simulink model "Multibody_model_El_winch"  (R2023b)
settings: Solver=FixedStepAuto  StartTime=0.0  StopTime=25  FixedStep=0.001  RelTol=1e-3
model workspace (MATLAB code in the model file):
  | % Parameters
  | Q_max = 130; %L/min |  2 vales w max 65 L/min
  | 
  | %Load Parameters
  | m_pl = 1000;
  | r_d = 0.035;
  | ig = 5;
  | J_drum = 0.0006125; % 1/2MR^2
  | b_hat = 0.001;
  | 
  | % Motor Parameters
  | np=2;
  | P_N = 15000;
  | n_eff = 0.917;
  | n_rpm = 1469;
  | pf = 0.84;
  | I_N = 29;
  | Is_In = 8;
  | T_n = 97.5;
  | Ti_Tn = 3.1;
  | Tb_Tn = 3.6;
  | J_motor = 0.13;
  | 
  | % Inv-Gamma Circuit parameters
  | 
  | R_R_hat = 0.2052;
  | X_M_opt = 15.1061;
  | X_sig_opt = 0.3774;
  | omega_rN = 307.6666;
  | omega_N = 314.1593;
  | omega1 = omega_rN;
  | L_M_hat = X_M_opt/omega1;
  | L_sig_hat = X_sig_opt/omega1;
  | R_s = 0.619;
  | 
  | 
  | psi_ref = 20*P_N/(sqrt(2)*pi*np*I_N*n_rpm);
  | 
  | % Others
  | V_base = 400*sqrt(2)/sqrt(3);
  | I_max = I_N*3;
  | 
  | % Speed Controller
  | t_r = 1e-3;
  | w_BW = log(9)/t_r;
  | w_BWs = 0.1*w_BW;
  | J_hat = m_pl*((r_d/(ig))^2) + J_drum*((1/ig)^2) + J_motor;
  | kps = 2*J_hat*w_BWs/(3*np^2*psi_ref);
  | kis = w_BWs^2*2*J_hat/(3*np^2*psi_ref);
  | Ba = 2*J_hat/(3*np^2*psi_ref)*(w_BWs-b_hat/J_hat);
  | 
  | % Current Controller
  | kp = w_BW*L_sig_hat;
  | ki = w_BW^2*L_sig_hat;
  | Ra = w_BW*L_sig_hat - (R_R_hat + R_s);
  | R = R_R_hat + R_s;
undefined symbols (not defined in the file or in its folder): j, magnitude, X, Y, Z
libraries: sm_lib x44, fl_lib x24, nesl_utility x22, SimscapeFluids_lib x8, slpidlib x4, spsRMSLib x1, simulink x1
(part 4 of 4)

== system Multibody_model_El_winch/Electrical Winch/Current Controller and Flux Estimator/IM/alphabeta->abc ==
  note: u(2)
  note: u(1)
  note: u(2)
  note: u(1)
  note: u(2)
  note: u(1)
  i_s^s : Inport
  Complex to Real-Imag : ComplexToRealImag
  Fcn : Fcn  Expr=u(1)
  Fcn1 : Fcn  Expr=-0.5*u(1)+0.5*sqrt(3)*u(2)
  Fcn2 : Fcn  Expr=-0.5*u(1)-0.5*sqrt(3)*u(2)
  Mux : Mux  Inputs=2
  Mux1 : Mux  Inputs=2
  Mux2 : Mux  Inputs=2
  Mux3 : Mux  Inputs=3
  is_abc : Outport
  wires:
  Mux3/1 -> is_abc/1
  Fcn2/1 -> Mux3/3
  Fcn1/1 -> Mux3/2
  Fcn/1 -> Mux3/1
  i_s^s/1 -> Complex to Real-Imag/1
  Mux2/1 -> Fcn2/1
  Mux1/1 -> Fcn1/1
  Complex to Real-Imag/2 -> Mux2/2, Mux1/2, Mux/2  "beta"
  Complex to Real-Imag/1 -> Mux2/1, Mux1/1, Mux/1  "alpha"
  Mux/1 -> Fcn/1

== system Multibody_model_El_winch/Electrical Winch/Current Controller and Flux Estimator/IM/Voltage Equations/Integrator (Complex Signal) ==
  u : Inport
  Complex to Real-Imag : ComplexToRealImag
  Integrator : Integrator  InitialCondition=psi_ref
  Integrator1 : Integrator
  Real-Imag to Complex : RealImagToComplex
  y : Outport
  wires:
  u/1 -> Complex to Real-Imag/1
  Real-Imag to Complex/1 -> y/1
  Integrator1/1 -> Real-Imag to Complex/2
  Integrator/1 -> Real-Imag to Complex/1
  Complex to Real-Imag/2 -> Integrator1/1
  Complex to Real-Imag/1 -> Integrator/1

== system Multibody_model_El_winch/Electrical Winch/Current Controller and Flux Estimator/IM/Voltage Equations/Integrator (Complex Signal)1 ==
  u : Inport
  Complex to Real-Imag : ComplexToRealImag
  Integrator : Integrator  InitialCondition=psi_ref
  Integrator1 : Integrator
  Real-Imag to Complex : RealImagToComplex
  y : Outport
  wires:
  u/1 -> Complex to Real-Imag/1
  Real-Imag to Complex/1 -> y/1
  Integrator1/1 -> Real-Imag to Complex/2
  Integrator/1 -> Real-Imag to Complex/1
  Complex to Real-Imag/2 -> Integrator1/1
  Complex to Real-Imag/1 -> Integrator/1

== matlab function Multibody_model_El_winch/Electrical Winch/Current Controller and Flux Estimator/dq->abc/MATLAB Function ==
  data: vs_dq input size=2; thetas input size=1; vs_abc output size=3
function vs_abc = dq_abc(vs_dq, thetas)
%#codegen

% voltage in synchronous coordinates:
 vd = vs_dq(1); vq = vs_dq(2); 
vs_dq = [vd;vq];

% coordinate transformation and Space-vector transformation 
T_alphabeta = [cos(thetas), -sin(thetas); sin(thetas), cos(thetas)];
T_23 = [1, 0; -1/2, sqrt(3)/2; -1/2, -sqrt(3)/2];
vs_abc = T_23*T_alphabeta*vs_dq;   % Complete this

== matlab function Multibody_model_El_winch/Hydraulic System/DCV_cylinder/MATLAB Function ==
  data: u input; pLS output; pA input; pB input
function pLS = fcn(u,pA,pB)
uEps = 0.05; %Deadband
if u < -uEps
    pLS = pB;
elseif u < uEps
    pLS = 0;
else
    pLS = pA;
end

== matlab function Multibody_model_El_winch/Hydraulic System/Pump/MATLAB Function ==
  data: u input; Q_Out output; Q_Max input
function Q_Out = fcn(u, Q_Max)

Q_Out = u*Q_Max/(60*10^3);

== matlab function Multibody_model_El_winch/Hydraulic System/Cylinder Control System/LoadCases, Cylinder ==
  data: cyl_sp output; sel input; Lc1_pos input; Lc2_pos input; Lc3_pos input; Lc1_vel input; Lc2_vel input; Lc3_vel input; cyl_vel output
function [cyl_sp, cyl_vel] = fcn(sel, Lc1_pos, Lc2_pos, Lc3_pos, Lc1_vel, Lc2_vel, Lc3_vel)

if sel == 1
    cyl_sp = Lc1_pos;
    cyl_vel = Lc1_vel;
elseif sel == 2
    cyl_sp = Lc2_pos;
    cyl_vel = Lc2_vel;
elseif sel == 3
    cyl_sp = Lc3_pos;
    cyl_vel = Lc3_vel;
else
    cyl_sp = 0;
    cyl_vel = 0; 
end

== matlab function Multibody_model_El_winch/Hydraulic System/Winch Control System/LoadCases, Cylinder ==
  data: winch_sp output; sel input; Lc1_pos input; Lc2_pos input; Lc3_pos input; Lc1_vel input; Lc2_vel input; Lc3_vel input; wich_vel output
function [winch_sp, wich_vel] = fcn(sel, Lc1_pos, Lc2_pos, Lc3_pos, Lc1_vel, Lc2_vel, Lc3_vel)

if sel == 1
    winch_sp = Lc1_pos;
    wich_vel = Lc1_vel;
elseif sel == 2
    winch_sp = Lc2_pos;
    wich_vel = Lc2_vel;
elseif sel == 3
    winch_sp = Lc3_pos;
    wich_vel = Lc3_vel;
else
    winch_sp = 0;
    wich_vel = 0; 
end

== matlab function Multibody_model_El_winch/Electrical Winch/Current Controller and Flux Estimator/Current Controller/MATLAB Function ==
  data: v_sat_dq input size=2; i_s_ref input size=2; i_s input size=2; w_1 input size=1; I input size=1; w_BW parameter size=1; v_s_ref output size=2; Inew output; R_R_hat parameter size=1; L_sig_hat parameter size=1; R_s input
function [v_s_ref, Inew] = cc(v_sat_dq,i_s_ref, i_s, w_1, I, w_BW, R_R_hat, L_sig_hat, R_s)
%#codegen

%% Current controller 
% Gains
Ts = 0.001;
kp = w_BW*L_sig_hat; % L7 p15
ki = w_BW^2*L_sig_hat; % L7 p15
Ra = w_BW*L_sig_hat - (R_R_hat + R_s); % L7 p14(R_R_hat+R_s)

% Voltage reference in synchronous coordinates
i_s = i_s(1)+ 1i*i_s(2);
i_s_ref = i_s_ref(1)+ 1i*i_s_ref(2);
e = i_s_ref - i_s;
% L7 p13 and p15 (c for complex number)
v_s_ref_c = kp*e+ki*I + 1i*w_1*L_sig_hat*i_s_ref-Ra*i_s_ref; % complete: PI + active resistance Ra + decoupler.
v_s_ref = [real(v_s_ref_c);imag(v_s_ref_c)];

%% Update the integral state of the current controller 
v_sat_dq_c = v_sat_dq(1)+ 1i*v_sat_dq(2);
Inew = I + Ts*(e + (v_sat_dq_c)/kp);

== matlab function Multibody_model_El_winch/Electrical Winch/Current Controller and Flux Estimator/abc->dq1/MATLAB Function ==
  data: is_abc input size=3; thetas input size=1; is output size=2
function is = abc_dq(is_abc, thetas)
%#codegen

% Phase currents
ia = is_abc(1); ib = is_abc(2); ic = is_abc(3); 
is_abc = [ia;ib;ic];
% Space-vector transformation and coordinate transformation
T_dq = [cos(thetas), sin(thetas); -sin(thetas), cos(thetas)];
T_32 = [2/3, -1/3, -1/3; 0, 1/sqrt(3), -1/sqrt(3)];
is = T_dq*T_32*is_abc;   % Complete this
